simulink library "rov_design_analysis"  (Simulink 6.0)
settings: Solver=ode45  SolverMode=SingleTasking  StartTime=0.0  StopTime=10.0  RelTol=1e-3
undefined symbols (not defined in the file or in its folder): amp, At, B, Bt, Ct, cycles, D, den, DL, Do, DQ, DQL, freq, frtest, I, L, m, M, Ma, magnitude, MaU, Mt, nmiss, num, phase, rg, sigbuilder_block, slcm, T, W, xb, xg, Xudot, yb, yg, Yvdot, zb, zg, Zwdot
libraries: simulink_extras x32, simulink x27, rov_design_analysis x15, marine_gnc x10, dspmtrx2 x6, dspstat3 x4
(part 9 of 9)

== system rov_design_analysis/ROV Controller /Nonlinear-Sliding-Mode Cascaded  Controller - 6 DoF/Body-fixed to Earth_fixed Transformation1/Transformation matrix R/Row2 of T/Dot Product1 ==
  in_1 : Inport  Port=1  LatchInput=off
  in_2 : Inport  Port=2  LatchInput=off
  Product : Product  SaturateOnIntegerOverflow=on  RndMeth=Zero  InputSameDT=on
  Sum : Sum  Inputs=+  SaturateOnIntegerOverflow=on  InputSameDT=on
  out_1 : Outport  InitialOutput=0
  wires:
  Sum/1 -> out_1/1
  Product/1 -> Sum/1
  in_1/1 -> Product/1
  in_2/1 -> Product/2

== system rov_design_analysis/ROV Controller /Nonlinear-Sliding-Mode Cascaded  Controller - 6 DoF/Body-fixed to Earth_fixed Transformation1/Transformation matrix R/Row3 of T/Dot Product1 ==
  in_1 : Inport  Port=1  LatchInput=off
  in_2 : Inport  Port=2  LatchInput=off
  Product : Product  SaturateOnIntegerOverflow=on  RndMeth=Zero  InputSameDT=on
  Sum : Sum  Inputs=+  SaturateOnIntegerOverflow=on  InputSameDT=on
  out_1 : Outport  InitialOutput=0
  wires:
  Sum/1 -> out_1/1
  Product/1 -> Sum/1
  in_1/1 -> Product/1
  in_2/1 -> Product/2

== system rov_design_analysis/ROV Controller /Nonlinear-Sliding-Mode Cascaded  Controller - 6 DoF/Body-fixed to Earth_fixed Transformation1/Transformation matrix T/Row1 of R/Dot Product ==
  in_1 : Inport  Port=1  LatchInput=off
  in_2 : Inport  Port=2  LatchInput=off
  Product : Product  SaturateOnIntegerOverflow=on  RndMeth=Zero  InputSameDT=on
  Sum : Sum  Inputs=+  SaturateOnIntegerOverflow=on  InputSameDT=on
  out_1 : Outport  InitialOutput=0
  wires:
  Sum/1 -> out_1/1
  Product/1 -> Sum/1
  in_1/1 -> Product/1
  in_2/1 -> Product/2

== system rov_design_analysis/ROV Controller /Nonlinear-Sliding-Mode Cascaded  Controller - 6 DoF/Body-fixed to Earth_fixed Transformation1/Transformation matrix T/Row2 of R/Dot Product1 ==
  in_1 : Inport  Port=1  LatchInput=off
  in_2 : Inport  Port=2  LatchInput=off
  Product : Product  SaturateOnIntegerOverflow=on  RndMeth=Zero  InputSameDT=on
  Sum : Sum  Inputs=+  SaturateOnIntegerOverflow=on  InputSameDT=on
  out_1 : Outport  InitialOutput=0
  wires:
  Sum/1 -> out_1/1
  Product/1 -> Sum/1
  in_1/1 -> Product/1
  in_2/1 -> Product/2

== system rov_design_analysis/ROV Controller /Nonlinear-Sliding-Mode Cascaded  Controller - 6 DoF/Body-fixed to Earth_fixed Transformation1/Transformation matrix T/Row3 of R/Dot Product1 ==
  in_1 : Inport  Port=1  LatchInput=off
  in_2 : Inport  Port=2  LatchInput=off
  Product : Product  SaturateOnIntegerOverflow=on  RndMeth=Zero  InputSameDT=on
  Sum : Sum  Inputs=+  SaturateOnIntegerOverflow=on  InputSameDT=on
  out_1 : Outport  InitialOutput=0
  wires:
  Sum/1 -> out_1/1
  Product/1 -> Sum/1
  in_1/1 -> Product/1
  in_2/1 -> Product/2

== system rov_design_analysis/ROV Controller /Nonlinear-Sliding-Mode Cascaded  Controller - 6 DoF/Body-fixed to Earth_fixed Transformation3/Transformation matrix R/Row1 of T/Dot Product1 ==
  in_1 : Inport  Port=1  LatchInput=off
  in_2 : Inport  Port=2  LatchInput=off
  Product : Product  SaturateOnIntegerOverflow=on  RndMeth=Zero  InputSameDT=on
  Sum : Sum  Inputs=+  SaturateOnIntegerOverflow=on  InputSameDT=on
  out_1 : Outport  InitialOutput=0
  wires:
  in_2/1 -> Product/2
  in_1/1 -> Product/1
  Product/1 -> Sum/1
  Sum/1 -> out_1/1

== system rov_design_analysis/ROV Controller /Nonlinear-Sliding-Mode Cascaded  Controller - 6 DoF/Body-fixed to Earth_fixed Transformation3/Transformation matrix R/Row2 of T/Dot Product1 ==
  in_1 : Inport  Port=1  LatchInput=off
  in_2 : Inport  Port=2  LatchInput=off
  Product : Product  SaturateOnIntegerOverflow=on  RndMeth=Zero  InputSameDT=on
  Sum : Sum  Inputs=+  SaturateOnIntegerOverflow=on  InputSameDT=on
  out_1 : Outport  InitialOutput=0
  wires:
  in_2/1 -> Product/2
  in_1/1 -> Product/1
  Product/1 -> Sum/1
  Sum/1 -> out_1/1

== system rov_design_analysis/ROV Controller /Nonlinear-Sliding-Mode Cascaded  Controller - 6 DoF/Body-fixed to Earth_fixed Transformation3/Transformation matrix R/Row3 of T/Dot Product1 ==
  in_1 : Inport  Port=1  LatchInput=off
  in_2 : Inport  Port=2  LatchInput=off
  Product : Product  SaturateOnIntegerOverflow=on  RndMeth=Zero  InputSameDT=on
  Sum : Sum  Inputs=+  SaturateOnIntegerOverflow=on  InputSameDT=on
  out_1 : Outport  InitialOutput=0
  wires:
  in_2/1 -> Product/2
  in_1/1 -> Product/1
  Product/1 -> Sum/1
  Sum/1 -> out_1/1

== system rov_design_analysis/ROV Controller /Nonlinear-Sliding-Mode Cascaded  Controller - 6 DoF/Body-fixed to Earth_fixed Transformation3/Transformation matrix T/Row1 of R/Dot Product ==
  in_1 : Inport  Port=1  LatchInput=off
  in_2 : Inport  Port=2  LatchInput=off
  Product : Product  SaturateOnIntegerOverflow=on  RndMeth=Zero  InputSameDT=on
  Sum : Sum  Inputs=+  SaturateOnIntegerOverflow=on  InputSameDT=on
  out_1 : Outport  InitialOutput=0
  wires:
  in_2/1 -> Product/2
  in_1/1 -> Product/1
  Product/1 -> Sum/1
  Sum/1 -> out_1/1

== system rov_design_analysis/ROV Controller /Nonlinear-Sliding-Mode Cascaded  Controller - 6 DoF/Body-fixed to Earth_fixed Transformation3/Transformation matrix T/Row2 of R/Dot Product1 ==
  in_1 : Inport  Port=1  LatchInput=off
  in_2 : Inport  Port=2  LatchInput=off
  Product : Product  SaturateOnIntegerOverflow=on  RndMeth=Zero  InputSameDT=on
  Sum : Sum  Inputs=+  SaturateOnIntegerOverflow=on  InputSameDT=on
  out_1 : Outport  InitialOutput=0
  wires:
  in_2/1 -> Product/2
  in_1/1 -> Product/1
  Product/1 -> Sum/1
  Sum/1 -> out_1/1

== system rov_design_analysis/ROV Controller /Nonlinear-Sliding-Mode Cascaded  Controller - 6 DoF/Body-fixed to Earth_fixed Transformation3/Transformation matrix T/Row3 of R/Dot Product1 ==
  in_1 : Inport  Port=1  LatchInput=off
  in_2 : Inport  Port=2  LatchInput=off
  Product : Product  SaturateOnIntegerOverflow=on  RndMeth=Zero  InputSameDT=on
  Sum : Sum  Inputs=+  SaturateOnIntegerOverflow=on  InputSameDT=on
  out_1 : Outport  InitialOutput=0
  wires:
  in_2/1 -> Product/2
  in_1/1 -> Product/1
  Product/1 -> Sum/1
  Sum/1 -> out_1/1

== system rov_design_analysis/ROV Controller /P-Decoupled  Cascaded loop Controller  - 6 DoF/Body-fixed to Earth_fixed Transformation1/Transformation matrix R/Row1 of T/Dot Product1 ==
  in_1 : Inport  Port=1  LatchInput=off
  in_2 : Inport  Port=2  LatchInput=off
  Product : Product  SaturateOnIntegerOverflow=on  RndMeth=Zero  InputSameDT=on
  Sum : Sum  Inputs=+  SaturateOnIntegerOverflow=on  InputSameDT=on
  out_1 : Outport  InitialOutput=0
  wires:
  Sum/1 -> out_1/1
  Product/1 -> Sum/1
  in_1/1 -> Product/1
  in_2/1 -> Product/2

== system rov_design_analysis/ROV Controller /P-Decoupled  Cascaded loop Controller  - 6 DoF/Body-fixed to Earth_fixed Transformation1/Transformation matrix R/Row2 of T/Dot Product1 ==
  in_1 : Inport  Port=1  LatchInput=off
  in_2 : Inport  Port=2  LatchInput=off
  Product : Product  SaturateOnIntegerOverflow=on  RndMeth=Zero  InputSameDT=on
  Sum : Sum  Inputs=+  SaturateOnIntegerOverflow=on  InputSameDT=on
  out_1 : Outport  InitialOutput=0
  wires:
  Sum/1 -> out_1/1
  Product/1 -> Sum/1
  in_1/1 -> Product/1
  in_2/1 -> Product/2

== system rov_design_analysis/ROV Controller /P-Decoupled  Cascaded loop Controller  - 6 DoF/Body-fixed to Earth_fixed Transformation1/Transformation matrix R/Row3 of T/Dot Product1 ==
  in_1 : Inport  Port=1  LatchInput=off
  in_2 : Inport  Port=2  LatchInput=off
  Product : Product  SaturateOnIntegerOverflow=on  RndMeth=Zero  InputSameDT=on
  Sum : Sum  Inputs=+  SaturateOnIntegerOverflow=on  InputSameDT=on
  out_1 : Outport  InitialOutput=0
  wires:
  Sum/1 -> out_1/1
  Product/1 -> Sum/1
  in_1/1 -> Product/1
  in_2/1 -> Product/2

== system rov_design_analysis/ROV Controller /P-Decoupled  Cascaded loop Controller  - 6 DoF/Body-fixed to Earth_fixed Transformation1/Transformation matrix T/Row1 of R/Dot Product ==
  in_1 : Inport  Port=1  LatchInput=off
  in_2 : Inport  Port=2  LatchInput=off
  Product : Product  SaturateOnIntegerOverflow=on  RndMeth=Zero  InputSameDT=on
  Sum : Sum  Inputs=+  SaturateOnIntegerOverflow=on  InputSameDT=on
  out_1 : Outport  InitialOutput=0
  wires:
  Sum/1 -> out_1/1
  Product/1 -> Sum/1
  in_1/1 -> Product/1
  in_2/1 -> Product/2

== system rov_design_analysis/ROV Controller /P-Decoupled  Cascaded loop Controller  - 6 DoF/Body-fixed to Earth_fixed Transformation1/Transformation matrix T/Row2 of R/Dot Product1 ==
  in_1 : Inport  Port=1  LatchInput=off
  in_2 : Inport  Port=2  LatchInput=off
  Product : Product  SaturateOnIntegerOverflow=on  RndMeth=Zero  InputSameDT=on
  Sum : Sum  Inputs=+  SaturateOnIntegerOverflow=on  InputSameDT=on
  out_1 : Outport  InitialOutput=0
  wires:
  Sum/1 -> out_1/1
  Product/1 -> Sum/1
  in_1/1 -> Product/1
  in_2/1 -> Product/2

== system rov_design_analysis/ROV Controller /P-Decoupled  Cascaded loop Controller  - 6 DoF/Body-fixed to Earth_fixed Transformation1/Transformation matrix T/Row3 of R/Dot Product1 ==
  in_1 : Inport  Port=1  LatchInput=off
  in_2 : Inport  Port=2  LatchInput=off
  Product : Product  SaturateOnIntegerOverflow=on  RndMeth=Zero  InputSameDT=on
  Sum : Sum  Inputs=+  SaturateOnIntegerOverflow=on  InputSameDT=on
  out_1 : Outport  InitialOutput=0
  wires:
  Sum/1 -> out_1/1
  Product/1 -> Sum/1
  in_1/1 -> Product/1
  in_2/1 -> Product/2

== system rov_design_analysis/ROV Controller /P-Decoupled  Cascaded loop Controller  - 6 DoF/Body-fixed to Earth_fixed Transformation3/Transformation matrix R/Row1 of T/Dot Product1 ==
  in_1 : Inport  Port=1  LatchInput=off
  in_2 : Inport  Port=2  LatchInput=off
  Product : Product  SaturateOnIntegerOverflow=on  RndMeth=Zero  InputSameDT=on
  Sum : Sum  Inputs=+  SaturateOnIntegerOverflow=on  InputSameDT=on
  out_1 : Outport  InitialOutput=0
  wires:
  in_2/1 -> Product/2
  in_1/1 -> Product/1
  Product/1 -> Sum/1
  Sum/1 -> out_1/1

== system rov_design_analysis/ROV Controller /P-Decoupled  Cascaded loop Controller  - 6 DoF/Body-fixed to Earth_fixed Transformation3/Transformation matrix R/Row2 of T/Dot Product1 ==
  in_1 : Inport  Port=1  LatchInput=off
  in_2 : Inport  Port=2  LatchInput=off
  Product : Product  SaturateOnIntegerOverflow=on  RndMeth=Zero  InputSameDT=on
  Sum : Sum  Inputs=+  SaturateOnIntegerOverflow=on  InputSameDT=on
  out_1 : Outport  InitialOutput=0
  wires:
  in_2/1 -> Product/2
  in_1/1 -> Product/1
  Product/1 -> Sum/1
  Sum/1 -> out_1/1

== system rov_design_analysis/ROV Controller /P-Decoupled  Cascaded loop Controller  - 6 DoF/Body-fixed to Earth_fixed Transformation3/Transformation matrix R/Row3 of T/Dot Product1 ==
  in_1 : Inport  Port=1  LatchInput=off
  in_2 : Inport  Port=2  LatchInput=off
  Product : Product  SaturateOnIntegerOverflow=on  RndMeth=Zero  InputSameDT=on
  Sum : Sum  Inputs=+  SaturateOnIntegerOverflow=on  InputSameDT=on
  out_1 : Outport  InitialOutput=0
  wires:
  in_2/1 -> Product/2
  in_1/1 -> Product/1
  Product/1 -> Sum/1
  Sum/1 -> out_1/1

== system rov_design_analysis/ROV Controller /P-Decoupled  Cascaded loop Controller  - 6 DoF/Body-fixed to Earth_fixed Transformation3/Transformation matrix T/Row1 of R/Dot Product ==
  in_1 : Inport  Port=1  LatchInput=off
  in_2 : Inport  Port=2  LatchInput=off
  Product : Product  SaturateOnIntegerOverflow=on  RndMeth=Zero  InputSameDT=on
  Sum : Sum  Inputs=+  SaturateOnIntegerOverflow=on  InputSameDT=on
  out_1 : Outport  InitialOutput=0
  wires:
  in_2/1 -> Product/2
  in_1/1 -> Product/1
  Product/1 -> Sum/1
  Sum/1 -> out_1/1

== system rov_design_analysis/ROV Controller /P-Decoupled  Cascaded loop Controller  - 6 DoF/Body-fixed to Earth_fixed Transformation3/Transformation matrix T/Row2 of R/Dot Product1 ==
  in_1 : Inport  Port=1  LatchInput=off
  in_2 : Inport  Port=2  LatchInput=off
  Product : Product  SaturateOnIntegerOverflow=on  RndMeth=Zero  InputSameDT=on
  Sum : Sum  Inputs=+  SaturateOnIntegerOverflow=on  InputSameDT=on
  out_1 : Outport  InitialOutput=0
  wires:
  in_2/1 -> Product/2
  in_1/1 -> Product/1
  Product/1 -> Sum/1
  Sum/1 -> out_1/1

== system rov_design_analysis/ROV Controller /P-Decoupled  Cascaded loop Controller  - 6 DoF/Body-fixed to Earth_fixed Transformation3/Transformation matrix T/Row3 of R/Dot Product1 ==
  in_1 : Inport  Port=1  LatchInput=off
  in_2 : Inport  Port=2  LatchInput=off
  Product : Product  SaturateOnIntegerOverflow=on  RndMeth=Zero  InputSameDT=on
  Sum : Sum  Inputs=+  SaturateOnIntegerOverflow=on  InputSameDT=on
  out_1 : Outport  InitialOutput=0
  wires:
  in_2/1 -> Product/2
  in_1/1 -> Product/1
  Product/1 -> Sum/1
  Sum/1 -> out_1/1

== system rov_design_analysis/ROV Controller /P-Decoupled  Single loop Controller - 6 DoF /Body-fixed to Earth_fixed Transformation1/Transformation matrix R/Row1 of T/Dot Product1 ==
  in_1 : Inport  Port=1  LatchInput=off
  in_2 : Inport  Port=2  LatchInput=off
  Product : Product  SaturateOnIntegerOverflow=on  RndMeth=Zero  InputSameDT=on
  Sum : Sum  Inputs=+  SaturateOnIntegerOverflow=on  InputSameDT=on
  out_1 : Outport  InitialOutput=0
  wires:
  in_2/1 -> Product/2
  in_1/1 -> Product/1
  Product/1 -> Sum/1
  Sum/1 -> out_1/1

== system rov_design_analysis/ROV Controller /P-Decoupled  Single loop Controller - 6 DoF /Body-fixed to Earth_fixed Transformation1/Transformation matrix R/Row2 of T/Dot Product1 ==
  in_1 : Inport  Port=1  LatchInput=off
  in_2 : Inport  Port=2  LatchInput=off
  Product : Product  SaturateOnIntegerOverflow=on  RndMeth=Zero  InputSameDT=on
  Sum : Sum  Inputs=+  SaturateOnIntegerOverflow=on  InputSameDT=on
  out_1 : Outport  InitialOutput=0
  wires:
  in_2/1 -> Product/2
  in_1/1 -> Product/1
  Product/1 -> Sum/1
  Sum/1 -> out_1/1

== system rov_design_analysis/ROV Controller /P-Decoupled  Single loop Controller - 6 DoF /Body-fixed to Earth_fixed Transformation1/Transformation matrix R/Row3 of T/Dot Product1 ==
  in_1 : Inport  Port=1  LatchInput=off
  in_2 : Inport  Port=2  LatchInput=off
  Product : Product  SaturateOnIntegerOverflow=on  RndMeth=Zero  InputSameDT=on
  Sum : Sum  Inputs=+  SaturateOnIntegerOverflow=on  InputSameDT=on
  out_1 : Outport  InitialOutput=0
  wires:
  in_2/1 -> Product/2
  in_1/1 -> Product/1
  Product/1 -> Sum/1
  Sum/1 -> out_1/1

== system rov_design_analysis/ROV Controller /P-Decoupled  Single loop Controller - 6 DoF /Body-fixed to Earth_fixed Transformation1/Transformation matrix T/Row1 of R/Dot Product ==
  in_1 : Inport  Port=1  LatchInput=off
  in_2 : Inport  Port=2  LatchInput=off
  Product : Product  SaturateOnIntegerOverflow=on  RndMeth=Zero  InputSameDT=on
  Sum : Sum  Inputs=+  SaturateOnIntegerOverflow=on  InputSameDT=on
  out_1 : Outport  InitialOutput=0
  wires:
  in_2/1 -> Product/2
  in_1/1 -> Product/1
  Product/1 -> Sum/1
  Sum/1 -> out_1/1

== system rov_design_analysis/ROV Controller /P-Decoupled  Single loop Controller - 6 DoF /Body-fixed to Earth_fixed Transformation1/Transformation matrix T/Row2 of R/Dot Product1 ==
  in_1 : Inport  Port=1  LatchInput=off
  in_2 : Inport  Port=2  LatchInput=off
  Product : Product  SaturateOnIntegerOverflow=on  RndMeth=Zero  InputSameDT=on
  Sum : Sum  Inputs=+  SaturateOnIntegerOverflow=on  InputSameDT=on
  out_1 : Outport  InitialOutput=0
  wires:
  in_2/1 -> Product/2
  in_1/1 -> Product/1
  Product/1 -> Sum/1
  Sum/1 -> out_1/1

== system rov_design_analysis/ROV Controller /P-Decoupled  Single loop Controller - 6 DoF /Body-fixed to Earth_fixed Transformation1/Transformation matrix T/Row3 of R/Dot Product1 ==
  in_1 : Inport  Port=1  LatchInput=off
  in_2 : Inport  Port=2  LatchInput=off
  Product : Product  SaturateOnIntegerOverflow=on  RndMeth=Zero  InputSameDT=on
  Sum : Sum  Inputs=+  SaturateOnIntegerOverflow=on  InputSameDT=on
  out_1 : Outport  InitialOutput=0
  wires:
  in_2/1 -> Product/2
  in_1/1 -> Product/1
  Product/1 -> Sum/1
  Sum/1 -> out_1/1

== system rov_design_analysis/ROV Controller /P-Decoupled  Single loop Controller - 6 DoF /Body-fixed to Earth_fixed Transformation3/Transformation matrix R/Row1 of T/Dot Product1 ==
  in_1 : Inport  Port=1  LatchInput=off
  in_2 : Inport  Port=2  LatchInput=off
  Product : Product  SaturateOnIntegerOverflow=on  RndMeth=Zero  InputSameDT=on
  Sum : Sum  Inputs=+  SaturateOnIntegerOverflow=on  InputSameDT=on
  out_1 : Outport  InitialOutput=0
  wires:
  Sum/1 -> out_1/1
  Product/1 -> Sum/1
  in_1/1 -> Product/1
  in_2/1 -> Product/2

== system rov_design_analysis/ROV Controller /P-Decoupled  Single loop Controller - 6 DoF /Body-fixed to Earth_fixed Transformation3/Transformation matrix R/Row2 of T/Dot Product1 ==
  in_1 : Inport  Port=1  LatchInput=off
  in_2 : Inport  Port=2  LatchInput=off
  Product : Product  SaturateOnIntegerOverflow=on  RndMeth=Zero  InputSameDT=on
  Sum : Sum  Inputs=+  SaturateOnIntegerOverflow=on  InputSameDT=on
  out_1 : Outport  InitialOutput=0
  wires:
  Sum/1 -> out_1/1
  Product/1 -> Sum/1
  in_1/1 -> Product/1
  in_2/1 -> Product/2

== system rov_design_analysis/ROV Controller /P-Decoupled  Single loop Controller - 6 DoF /Body-fixed to Earth_fixed Transformation3/Transformation matrix R/Row3 of T/Dot Product1 ==
  in_1 : Inport  Port=1  LatchInput=off
  in_2 : Inport  Port=2  LatchInput=off
  Product : Product  SaturateOnIntegerOverflow=on  RndMeth=Zero  InputSameDT=on
  Sum : Sum  Inputs=+  SaturateOnIntegerOverflow=on  InputSameDT=on
  out_1 : Outport  InitialOutput=0
  wires:
  Sum/1 -> out_1/1
  Product/1 -> Sum/1
  in_1/1 -> Product/1
  in_2/1 -> Product/2

== system rov_design_analysis/ROV Controller /P-Decoupled  Single loop Controller - 6 DoF /Body-fixed to Earth_fixed Transformation3/Transformation matrix T/Row1 of R/Dot Product ==
  in_1 : Inport  Port=1  LatchInput=off
  in_2 : Inport  Port=2  LatchInput=off
  Product : Product  SaturateOnIntegerOverflow=on  RndMeth=Zero  InputSameDT=on
  Sum : Sum  Inputs=+  SaturateOnIntegerOverflow=on  InputSameDT=on
  out_1 : Outport  InitialOutput=0
  wires:
  Sum/1 -> out_1/1
  Product/1 -> Sum/1
  in_1/1 -> Product/1
  in_2/1 -> Product/2

== system rov_design_analysis/ROV Controller /P-Decoupled  Single loop Controller - 6 DoF /Body-fixed to Earth_fixed Transformation3/Transformation matrix T/Row2 of R/Dot Product1 ==
  in_1 : Inport  Port=1  LatchInput=off
  in_2 : Inport  Port=2  LatchInput=off
  Product : Product  SaturateOnIntegerOverflow=on  RndMeth=Zero  InputSameDT=on
  Sum : Sum  Inputs=+  SaturateOnIntegerOverflow=on  InputSameDT=on
  out_1 : Outport  InitialOutput=0
  wires:
  Sum/1 -> out_1/1
  Product/1 -> Sum/1
  in_1/1 -> Product/1
  in_2/1 -> Product/2

== system rov_design_analysis/ROV Controller /P-Decoupled  Single loop Controller - 6 DoF /Body-fixed to Earth_fixed Transformation3/Transformation matrix T/Row3 of R/Dot Product1 ==
  in_1 : Inport  Port=1  LatchInput=off
  in_2 : Inport  Port=2  LatchInput=off
  Product : Product  SaturateOnIntegerOverflow=on  RndMeth=Zero  InputSameDT=on
  Sum : Sum  Inputs=+  SaturateOnIntegerOverflow=on  InputSameDT=on
  out_1 : Outport  InitialOutput=0
  wires:
  Sum/1 -> out_1/1
  Product/1 -> Sum/1
  in_1/1 -> Product/1
  in_2/1 -> Product/2
